simulink model "validate_driving_mode"  (R2015a)
settings: Solver=ode45  StartTime=0.0  StopTime=10.0  RelTol=1e-3
undefined symbols (not defined in the file): sigbuilder_block
settings Model: Creator=Piyush  LastModifiedBy=Piyush

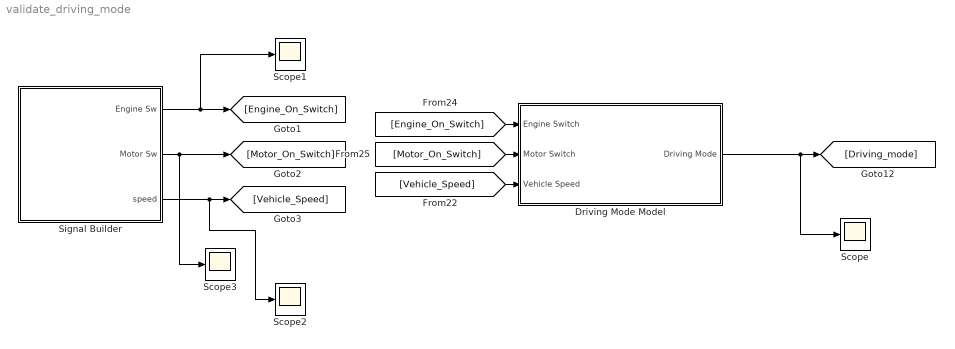
== system validate_driving_mode ==
  Driving Mode Model : Subsystem
  Scope{,1..3} (4 alike) : Scope
      Scope2 settings: SaveName=ScopeData2
      Scope3 settings: SaveName=ScopeData3
  Signal Builder : Subsystem  Tag=STV Subsys  LoadFcn=sigbuilder_block('load');  StartFcn=sigbuilder_block('start');  StopFcn=sigbuilder_block('stop');  ClipboardFcn=sigbuilder_block('clipboard');  mask(Sigbuilder block){}
      mask help: Simulink:masks:SigbuilderBlock_MD
      mask init:
      | if ~strcmp(get_param(bdroot(gcbh),'SimulationStatus'),'stopped') tuvar = sigbuilder_block('maskInit'); end
      settings: CopyFcn=sigbuilder_block('copy');  DeleteFcn=sigbuilder_block('delete');  ModelCloseFcn=sigbuilder_block('modelClose');  PreSaveFcn=sigbuilder_block('preSave');  PauseFcn=sigbuilder_block('pause');  ContinueFcn=sigbuilder_block('continue');  NameChangeFcn=sigbuilder_block('namechange');  OpenFcn=sigbuilder_block('open',[437.6 199.2 550.4 400 ]);  CloseFcn=sigbuilder_block('close');
      mask Display: plot(0, 0, 100, 100,[2, 2, 32, 32, 2], [68, 8, 8, 68, 68],[32, 2], [38, 38], [32, 19, 2],[53, 60, 44], [32, 17, 17, 2],[16, 16, 31, 31]);txt = getActiveGroup(gcbh);text(2, 100, txt,'verticalAlignment', 'top');
  wires:
  [Vehicle_Speed] -> Driving Mode Model/3(Vehicle Speed)
  [Engine_On_Switch] -> Driving Mode Model/1(Engine Switch)
  [Motor_On_Switch] -> Driving Mode Model/2(Motor Switch)
  Signal Builder/1(Engine Sw) -> Scope1/1, [Engine_On_Switch]
  Signal Builder/2(Motor Sw) -> Scope3/1, [Motor_On_Switch]
  Signal Builder/3(speed) -> Scope2/1, [Vehicle_Speed]
  Driving Mode Model/1(Driving Mode) -> Scope/1, [Driving_mode]

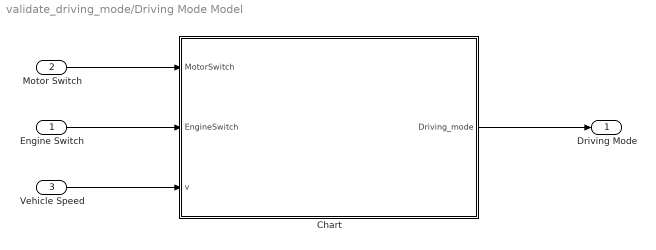
== system validate_driving_mode/Driving Mode Model ==
  Engine Switch : Inport
  Motor Switch : Inport  Port=2
  Vehicle Speed : Inport  Port=3
  Chart : Stateflow chart  TreatAsAtomicUnit=on
  Driving Mode : Outport
  wires:
  Motor Switch/1 -> Chart/1(MotorSwitch)
  Engine Switch/1 -> Chart/2(EngineSwitch)
  Vehicle Speed/1 -> Chart/3(v)
  Chart/1(Driving_mode) -> Driving Mode/1

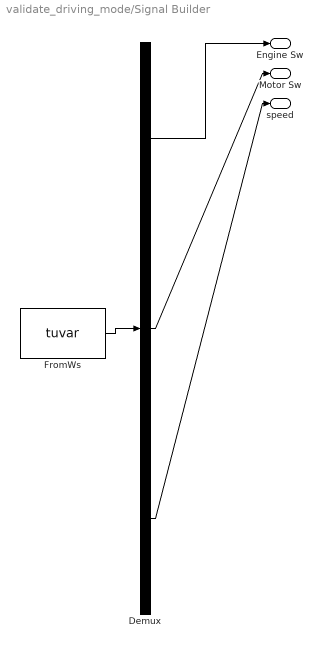
== system validate_driving_mode/Signal Builder ==
  Demux : Demux  Tag=STV Demux  Outputs=3
  FromWs : FromWorkspace  Tag=STV FromWs  VariableName=tuvar  SampleTime=0
      SigBuilderData=|
      | common.afterFinalStr = 'Extrapolate'
      | common.sampleTime = 0
      | dataSet.timeRange = [0 10]
      | dataSet.name = 'Group 1'
      | sbobj.Groups.Name = 'Group 1'
      | sbobj.Groups.Signals(1).Name = 'Engine Sw'
      | sbobj.Groups.Signals(1).XData = [0 1.01 1.01 1.99 6 6 10]
      | sbobj.Groups.Signals(1).YData = [0 0 1 1 1 0 0]
      | sbobj.Groups.Signals(2).Name = 'Motor Sw'
      | sbobj.Groups.Signals(2).XData = [0 1.14 1.14 2 2 7.44 7.44 10]
      | sbobj.Groups.Signals(2).YData = [1 1 0 0 1 1 0 0]
      | sbobj.Groups.Signals(3).Name = 'speed'
      | sbobj.Groups.Signals(3).XData = [0 0.99 1.32 1.48 1.99 2.49 2.49 3.13 4.78 4.78 10]
      | sbobj.Groups.Signals(3).YData = [0 1.17 1.1677385159 0 1.21 1.35 1.34 0 0 1.28 0]
  Engine Sw : Outport  Tag=STV Outport
  Motor Sw : Outport  Tag=STV Outport  Port=2
  speed : Outport  Tag=STV Outport  Port=3
  wires:
  Demux/1 -> Engine Sw/1
  FromWs/1 -> Demux/1
  Demux/2 -> Motor Sw/1
  Demux/3 -> speed/1

== stateflow chart validate_driving_mode/Driving Mode Model/Chart ==
  state Electric_solo_mode
    entry:Driving_mode=1;
    during:Driving_mode=1;
  state Blending_mode
    entry:Driving_mode=2;
    during:Driving_mode=2;
  state Engine_Solo_mode
    entry:Driving_mode=3;
    during: Driving_mode=3;
  (junction 12) -> Electric_solo_mode [order 2] : [MotorSwitch==1&&EngineSwitch==0&&v<1]
  Electric_solo_mode -> (junction 12) : [MotorSwitch==0&&v<1]
  (junction 12) -> Blending_mode [order 3] : [EngineSwitch==0&&MotorSwitch==0&&v<1]
  Blending_mode -> (junction 12) : [EngineSwitch==0||MotorSwitch==0&&v<1]
  (default) -> (junction 12)
  Engine_Solo_mode -> (junction 12) : [EngineSwitch==0&&v<1]
  (junction 12) -> Engine_Solo_mode [order 1] : [EngineSwitch==1&&MotorSwitch==0&&v<1]
  data: MotorSwitch input; EngineSwitch input; v input; Driving_mode output
